simulink model "two_link_model_active_compliance"  (R2021a)
settings: Solver=VariableStepAuto  StartTime=0.0  StopTime=100  RelTol=1e-3
undefined symbols (not defined in the file): a_1, a_2, F, K, K_D, K_P, o_r
settings Model: Creator=frida  LastModifiedBy=frida

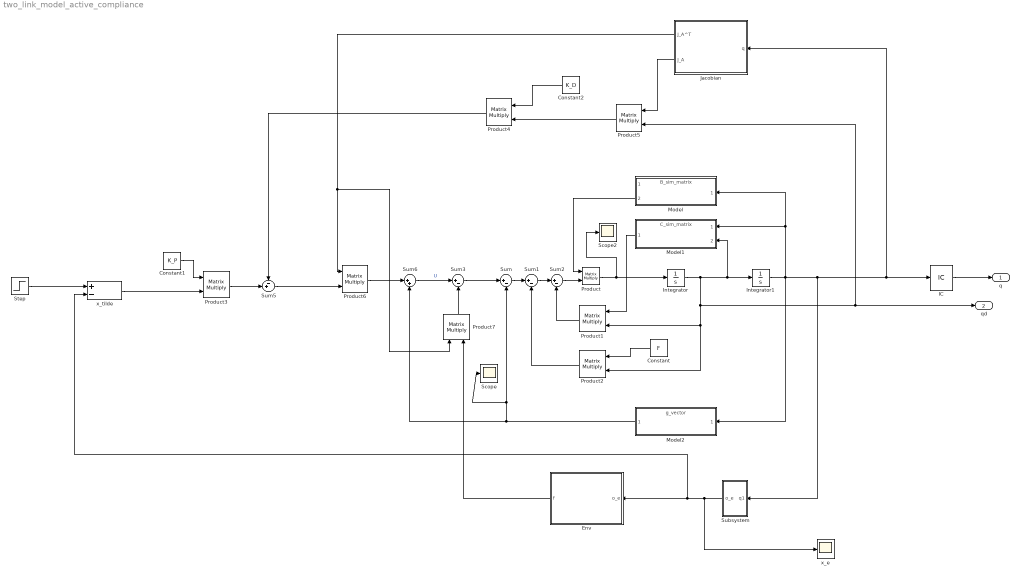
== system two_link_model_active_compliance ==
  Constant : Constant  Value=F
  Constant1 : Constant  Value=K_P
  Constant2 : Constant  Value=K_D
  Env : Subsystem
  IC : InitialCondition  Value=[0.75*pi, -0.75*pi]
  Integrator : Integrator
  Integrator1 : Integrator
  Jacobian : Subsystem
  Model : ModelReference  ModelNameDialog=B_sim_matrix.slx  SimulationMode=Normal  ModelReferenceVersion=1.6
  Model1 : ModelReference  ModelNameDialog=C_sim_matrix.slx  SimulationMode=Normal  ModelReferenceVersion=1.2
  Model2 : ModelReference  ModelNameDialog=g_vector.slx  SimulationMode=Normal  ModelReferenceVersion=1.8
  Product{,1..7} (8 alike) : Product  Multiplication=Matrix(*)
  Scope : Scope
  Scope2 : Scope
  Step : Step  After=[0.75;0.25];  SampleTime=0
  Subsystem : Subsystem
  Sum{,1..3} (4 alike) : Sum  Inputs=|+-
  Sum5 : Sum  Inputs=-+|
  Sum6 : Sum  Inputs=|++
  x_e : Scope
  x_tilde : Sum  Inputs=+-
  q : Outport  PortDimensions=2
  qd : Outport  Port=2  PortDimensions=2
  wires:
  Product3/1 -> Sum5/2
  Product/1 -> Scope2/1, Integrator/1
  Model2/1 -> Sum6/2, Scope/1, Sum/2
  Sum2/1 -> Product/2
  Product1/1 -> Sum2/2
  Integrator/1 -> qd/1, Product5/2, Product2/2, Product1/2, Model1/2, Integrator1/1
  Model/2 -> Product/1
  Product4/1 -> Sum5/1
  Integrator1/1 -> Model2/1, Subsystem/1(q1), Jacobian/1(q), IC/1, Model/1, Model1/1
  Sum/1 -> Sum1/1
  Model1/1 -> Product1/1
  Product2/1 -> Sum1/2
  Sum1/1 -> Sum2/1
  Constant/1 -> Product2/1
  Constant1/1 -> Product3/1
  Sum3/1 -> Sum/1
  Constant2/1 -> Product4/1
  Subsystem/1(o_e) -> x_e/1, x_tilde/2, Env/1(o_e)
  x_tilde/1 -> Product3/2
  Jacobian/2(J_A) -> Product5/1
  Product5/1 -> Product4/2
  Sum5/1 -> Product6/2
  Product6/1 -> Sum6/1
  Sum6/1 -> Sum3/1  "U"
  IC/1 -> q/1
  Env/1(f) -> Product7/2
  Product7/1 -> Sum3/2
  Jacobian/1(J_A^T) -> Product6/1, Product7/1
  Step/1 -> x_tilde/1

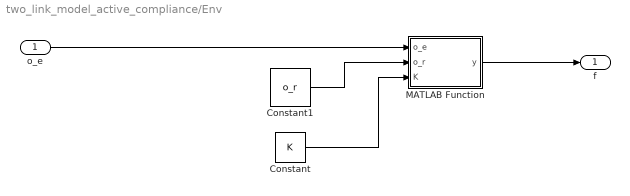
== system two_link_model_active_compliance/Env ==
  o_e : Inport
  Constant : Constant  Value=K
  Constant1 : Constant  Value=o_r
  MATLAB Function : MATLAB Function  TreatAsAtomicUnit=on
  f : Outport
  wires:
  Constant1/1 -> MATLAB Function/2(o_r)
  Constant/1 -> MATLAB Function/3(K)
  MATLAB Function/1(y) -> f/1
  o_e/1 -> MATLAB Function/1(o_e)

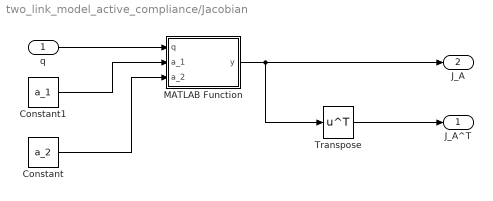
== system two_link_model_active_compliance/Jacobian ==
  q : Inport
  Constant : Constant  Value=a_2
  Constant1 : Constant  Value=a_1
  MATLAB Function : MATLAB Function  TreatAsAtomicUnit=on
  Transpose : Math  Operator=transpose  SaturateOnIntegerOverflow=on
  J_A^T : Outport
  J_A : Outport  Port=2
  wires:
  MATLAB Function/1(y) -> Transpose/1, J_A/1
  q/1 -> MATLAB Function/1(q)
  Constant1/1 -> MATLAB Function/2(a_1)
  Constant/1 -> MATLAB Function/3(a_2)
  Transpose/1 -> J_A^T/1

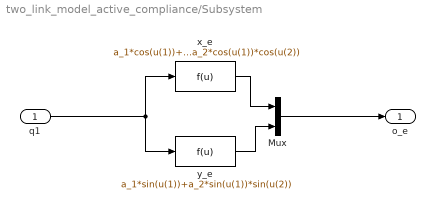
== system two_link_model_active_compliance/Subsystem ==
  q1 : Inport
  Mux : Mux  Inputs=2
  x_e : Fcn  Expr=a_1*cos(u(1))+a_2*cos(u(1))*cos(u(2))
  y_e : Fcn  Expr=a_1*sin(u(1))+a_2*sin(u(1))*sin(u(2))
  o_e : Outport
  wires:
  x_e/1 -> Mux/1
  Mux/1 -> o_e/1
  y_e/1 -> Mux/2
  q1/1 -> y_e/1, x_e/1

== matlab function two_link_model_active_compliance/Env/MATLAB Function ==
  data: o_e input; y output; o_r input; K input
function y = fcn(o_e, o_r, K)
if o_e(1) < o_r(1)
    y = [0; 0];
else
    % In this case the K matrix is a 
    % (2 x 2) matrix where only k_x is defined, 
    % therefore the returned y contains 
    % only forces in x-direction
    y = K*[o_e(1)-o_r(1); o_e(2)-o_r(2)];
end

== matlab function two_link_model_active_compliance/Jacobian/MATLAB Function ==
  data: q input; y output; a_1 input; a_2 input
function y = fcn(q, a_1, a_2)
y = [-a_1*sin(q(1)) - a_2*sin(q(1))*sin(q(2)), -a_2*sin(q(1))*sin(q(2));
    a_1*cos(q(1)) + a_2*cos(q(1))*cos(q(2)), a_2*cos(q(1))*cos(q(2))];
